simulink model "bandwidth_position"  (R2020b)
settings: Solver=ode4  StartTime=0.0  StopTime=10  FixedStep=1e-5  MaxStep=1e-4  RelTol=1e-4  EnableMultiTasking=on
values from neighbouring files (symbols this model uses):
  D = 0.1    [bandwidth.m]    (also in bandwidth_reference.m = 0.2; frequency_max_modulation_force.m = 0.9; frequency_max_modulation_force_sea.m = 0.9; frequency_max_modulation_position.m = 0.9)
  dm = 0.0068    [bandwidth.m]    (also in bandwidth_reference.m; frequency_max_modulation_force.m; frequency_max_modulation_force_sea.m; frequency_max_modulation_position.m)
  gear = 103    [bandwidth_reference.m]    (also in frequency_max_position.m; frequency_max_velocity.m; frequency_position.m; frequency_velocity.m)
  Jm = 0.0064    [bandwidth.m]    (also in bandwidth_reference.m = 0.0104; frequency_max_modulation_force.m = 0.0104; frequency_max_modulation_force_sea.m = 0.0104; frequency_max_modulation_position.m = 0.0104)
  kt = 1.5038    [bandwidth_reference.m]    (also in frequency_max_modulation_force.m; frequency_max_modulation_force_sea.m; frequency_max_modulation_position.m; frequency_max_modulation_velocity.m)
  P = 15    [bandwidth.m]    (also in bandwidth_reference.m = 1; frequency_max_modulation_force.m = 10; frequency_max_modulation_force_sea.m = 10; frequency_max_modulation_position.m = 10)
settings Model: Creator=eldisondimo  LastModifiedBy=filippo
settings DataIOCC: LimitDataPoints=on  SaveOutput=off  SaveTime=off  ReturnWorkspaceOutputs=off
settings OptimizationCC: ExpressionDepthLimit=2147483647  LifeSpan=1
settings DebuggingCC: UnderspecifiedInitializationDetection=Classic  MergeDetectMultiDrivingBlocksExec=none  FcnCallInpInsideContextMsg=warning  AllowSymbolicDim=off  StateNameClashWarn=warning  SFUnexpectedBacktrackingDiag=warning  SFNoUnconditionalDefaultTransitionDiag=warning  SFExecutionAtInitializationDiag=none  ArithmeticOperatorsInVariantConditions=warning
settings SFSimCC: SimUseLocalCustomCode=off  CustomCodeUndefinedFunction=UseInterfaceOnly
settings RTWCC: RTWUseLocalCustomCode=off
settings CodeAppCC: StateflowObjectComments=on
settings GRTTargetCC: TargetLangStandard=C89/C90 (ANSI)  CombineOutputUpdateFcns=off  GRTInterface=on

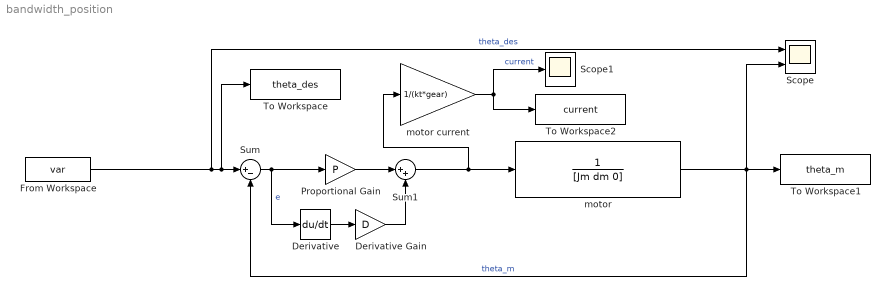
== system bandwidth_position ==
  Derivative : Derivative
  Derivative Gain : Gain  Gain=D
  From Workspace : FromWorkspace  VariableName=var
  Proportional Gain : Gain  Gain=P
  Scope : Scope  NumInputPorts=2
  Scope1 : Scope
  Sum : Sum  Inputs=|+-
  Sum1 : Sum  Inputs=|++
  To Workspace : ToWorkspace  VariableName=theta_des  SaveFormat=Structure With Time  SampleTime=-1
  To Workspace1 : ToWorkspace  VariableName=theta_m  SaveFormat=Structure With Time  SampleTime=-1
  To Workspace2 : ToWorkspace  VariableName=current  SaveFormat=Structure With Time  SampleTime=-1
  "motor " : TransferFcn  Denominator=[Jm dm 0]
  motor current : Gain  Gain=1/(kt*gear)
  wires:
  Sum/1 -> Proportional Gain/1, Derivative/1  "e"
  From Workspace/1 -> Scope/1, To Workspace/1, Sum/1  "theta_des"
  "motor "/1 -> Scope/2, To Workspace1/1, Sum/2  "theta_m"
  Proportional Gain/1 -> Sum1/1
  Derivative Gain/1 -> Sum1/2
  Derivative/1 -> Derivative Gain/1
  Sum1/1 -> motor current/1, "motor "/1
  motor current/1 -> Scope1/1, To Workspace2/1  "current"
